simulink model "OpenLoopLinearSimulink"  (R2023a)
settings: Solver=VariableStepAuto  StartTime=0.0  StopTime=14  RelTol=1e-3
values from neighbouring files (symbols this model uses):
  contrDerivs = [-0.166531614792 0.0128973723454 19.613884709 0 0 15.5648221946 0 0 0.0210537390355 -0.0037893723417 -0.882539324975 9.80664666251 ... (1248 elements, 48x26)]    [contrDerivs.mat]
  V_vals = [1, 5, 10, 15, 20, 25, 30, 35, 40, 45, 50, 55, 60, 65,      70, 75, 80, 85, 90, 95, 100, 105, 110, 115, 120, 125]    [coaxial_heli_parameters.m]    (also in initializeCCH.m = [1, 5, 10, 15, 20, 25, 30, 35, 40, 45, 50, 55, 60, 65,      )
  ytrim = ytrim(:,ii)    [initLinCCH6dof.m]
undefined symbols (not defined in the file or in its folder): stabDerivs
libraries: simulink_extras x3, cstblocks x1
settings Model: Creator=prenc  LastModifiedBy=prenc

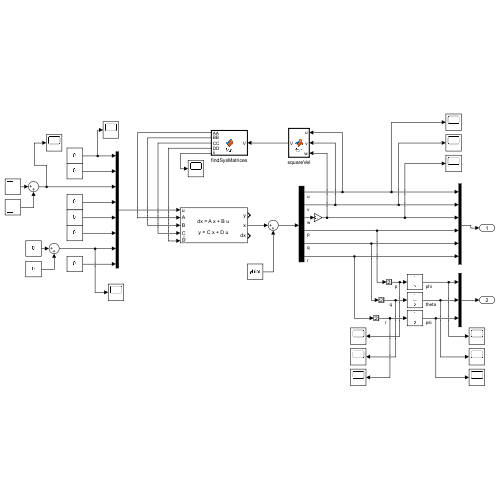
[thumbnail: Simulink's stored preview of the top-level diagram]
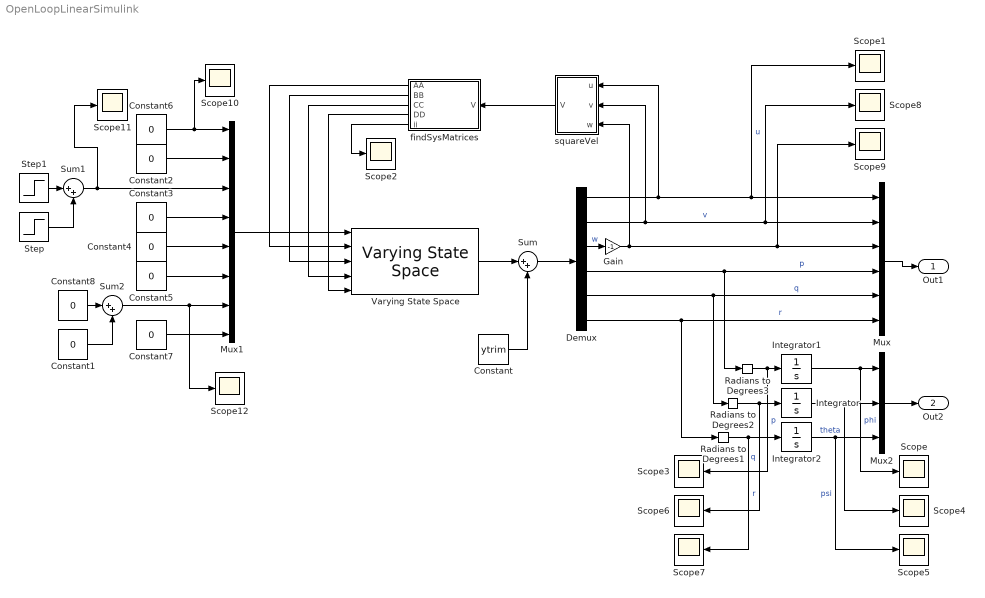
== system OpenLoopLinearSimulink ==
  Constant : Constant  Value=ytrim
  Constant{1..8} (8 alike) : Constant  Value=0
  Demux : Demux  Outputs=6
  Gain : Gain  Gain=-1
  Integrator : Integrator
  Integrator1 : Integrator
  Integrator2 : Integrator
  Mux : Mux  Inputs=6
  Mux1 : Mux  Inputs=8
  Mux2 : Mux  Inputs=3
  Radians to Degrees1 : simulink_extras/Transformations/Radians to Degrees
  Radians to Degrees2 : simulink_extras/Transformations/Radians to Degrees
  Radians to Degrees3 : simulink_extras/Transformations/Radians to Degrees
  Scope{,1..12} (13 alike) : Scope
  Step : Step  Time=4  After=deg2rad(1)  SampleTime=0
  Step1 : Step  Time=4.5  After=deg2rad(-1)  SampleTime=0
  Sum : Sum  Inputs=|++
  Sum1 : Sum  Inputs=|++
  Sum2 : Sum  Inputs=|++
  Varying State Space : cstblocks/Linear Parameter Varying/Varying State Space  x0=0  xNames=''  OutputX=on  OutputDX=on  Feedthrough=on
  findSysMatrices : MATLAB Function  TreatAsAtomicUnit=on
  squareVel : MATLAB Function  TreatAsAtomicUnit=on
  Out1 : Outport
  Out2 : Outport  Port=2
  wires:
  Demux/3 -> Gain/1  "w"
  Constant/1 -> Sum/2
  Demux/4 -> Radians to Degrees3/1, Mux/4  "p"
  Integrator2/1 -> Scope5/1, Mux2/3  "psi"
  Sum/1 -> Demux/1
  Demux/5 -> Radians to Degrees2/1, Mux/5  "q"
  Mux2/1 -> Out2/1
  Demux/2 -> Scope8/1, Mux/2, squareVel/2(v)  "v"
  Mux/1 -> Out1/1
  Mux1/1 -> Varying State Space/1
  Integrator/1 -> Scope4/1, Mux2/2  "theta"
  Demux/6 -> Radians to Degrees1/1, Mux/6  "r"
  Demux/1 -> Scope1/1, Mux/1, squareVel/1(u)  "u"
  Integrator1/1 -> Scope/1, Mux2/1  "phi"
  Constant6/1 -> Scope10/1, Mux1/1
  Constant2/1 -> Mux1/2
  Constant3/1 -> Mux1/4
  Constant4/1 -> Mux1/5
  Constant5/1 -> Mux1/6
  Sum2/1 -> Scope12/1, Mux1/7
  Constant7/1 -> Mux1/8
  Sum1/1 -> Scope11/1, Mux1/3
  Radians to Degrees2/1 -> Scope6/1, Integrator/1  "q"
  Radians to Degrees1/1 -> Scope7/1, Integrator2/1  "r"
  Radians to Degrees3/1 -> Scope3/1, Integrator1/1  "p"
  squareVel/1(V) -> findSysMatrices/1(V)
  findSysMatrices/2(BB) -> Varying State Space/3
  findSysMatrices/3(CC) -> Varying State Space/4
  findSysMatrices/4(DD) -> Varying State Space/5
  findSysMatrices/5(ii) -> Scope2/1
  findSysMatrices/1(AA) -> Varying State Space/2
  Varying State Space/2 -> Sum/1
  Gain/1 -> Scope9/1, Mux/3, squareVel/3(w)
  Constant1/1 -> Sum2/2
  Constant8/1 -> Sum2/1
  Step/1 -> Sum1/2
  Step1/1 -> Sum1/1

== matlab function OpenLoopLinearSimulink/squareVel ==
  data: u input; V output; v input; w input; trimvelocity parameter
function V = fcn(u,v,w, trimvelocity)

V = sqrt(u^2+v^2+w^2);

== matlab function OpenLoopLinearSimulink/findSysMatrices ==
  data: V input; AA output; BB output; CC output; DD output; V_vals parameter; stabDerivs parameter; contrDerivs parameter; ii output
function [AA, BB, CC, DD, ii] = fcn(V, V_vals, stabDerivs, contrDerivs)

    [~, ii] = min(abs(V_vals - V));
   

    X_u = stabDerivs(1,:); X_v = stabDerivs(2,:); X_w = stabDerivs(3,:); X_p = stabDerivs(4,:); X_q = stabDerivs(5,:); X_r = stabDerivs(6,:);
    Y_u = stabDerivs(7,:); Y_v = stabDerivs(8,:); Y_w = stabDerivs(9,:); Y_p = stabDerivs(10,:); Y_q = stabDerivs(11,:); Y_r = stabDerivs(12,:);
    Z_u = stabDerivs(13,:); Z_v = stabDerivs(14,:); Z_w = stabDerivs(15,:); Z_p = stabDerivs(16,:); Z_q = stabDerivs(17,:); Z_r = stabDerivs(18,:);
    L_u = stabDerivs(19,:); L_v = stabDerivs(20,:); L_w = stabDerivs(21,:); L_p = stabDerivs(22,:); L_q = stabDerivs(23,:); L_r = stabDerivs(24,:);
    M_u = stabDerivs(25,:); M_v = stabDerivs(26,:); M_w = stabDerivs(27,:); M_p = stabDerivs(28,:); M_q = stabDerivs(29,:); M_r = stabDerivs(30,:);
    N_u = stabDerivs(31,:); N_v = stabDerivs(32,:); N_w = stabDerivs(33,:); N_p = stabDerivs(34,:); N_q = stabDerivs(35,:); N_r = stabDerivs(36,:);

    
    AA = [X_u(ii), X_v(ii), X_w(ii), X_p(ii), X_q(ii), X_r(ii);
            Y_u(ii), Y_v(ii), Y_w(ii), Y_p(ii), Y_q(ii), Y_r(ii);
            Z_u(ii), Z_v(ii), Z_w(ii), Z_p(ii), Z_q(ii), Z_r(ii);
            L_u(ii), L_v(ii), L_w(ii), L_p(ii), L_q(ii), L_r(ii);
            M_u(ii), M_v(ii), M_w(ii), M_p(ii), M_q(ii), M_r(ii);
            N_u(ii), N_v(ii), N_w(ii), N_p(ii), N_q(ii), N_r(ii)];
    
    X_theta_0 = contrDerivs(1,:); X_theta_d = contrDerivs(2,:); X_theta_s = contrDerivs(3,:); X_theta_c = contrDerivs(4,:); X_theta_cdiff = contrDerivs(5,:); X_theta_p = contrDerivs(6,:); X_delta_e = contrDerivs(7,:); X_delta_r = contrDerivs(8,:);
    Y_theta_0 = contrDerivs(9,:); Y_theta_d = contrDerivs(10,:); Y_theta_s = contrDerivs(11,:); Y_theta_c = contrDerivs(12,:); Y_theta_cdiff = contrDerivs(13,:); Y_theta_p = contrDerivs(14,:); Y_delta_e = contrDerivs(15,:); Y_delta_r = contrDerivs(16,:);
    Z_theta_0 = contrDerivs(17,:); Z_theta_d = contrDerivs(18,:); Z_theta_s = contrDerivs(19,:); Z_theta_c = contrDerivs(20,:); Z_theta_cdiff = contrDerivs(21,:); Z_theta_p = contrDerivs(22,:); Z_delta_e = contrDerivs(23,:); Z_delta_r = contrDerivs(24,:);
    L_theta_0 = contrDerivs(25,:); L_theta_d = contrDerivs(26,:); L_theta_s = contrDerivs(27,:); L_theta_c = contrDerivs(28,:); L_theta_cdiff = contrDerivs(29,:); L_theta_p = contrDerivs(30,:); L_delta_e = contrDerivs(31,:); L_delta_r = contrDerivs(32,:);
    M_theta_0 = contrDerivs(33,:); M_theta_d = contrDerivs(34,:); M_theta_s = contrDerivs(35,:); M_theta_c = contrDerivs(36,:); M_theta_cdiff = contrDerivs(37,:); M_theta_p = contrDerivs(38,:); M_delta_e = contrDerivs(39,:); M_delta_r = contrDerivs(40,:);
    N_theta_0 = contrDerivs(41,:); N_theta_d = contrDerivs(42,:); N_theta_s = contrDerivs(43,:); N_theta_c = contrDerivs(44,:); N_theta_cdiff = contrDerivs(45,:); N_theta_p = contrDerivs(46,:); N_delta_e = contrDerivs(47,:); N_delta_r = contrDerivs(48,:);

    BB = [X_theta_0(ii), X_theta_d(ii), X_theta_s(ii), X_theta_c(ii), X_theta_cdiff(ii), X_theta_p(ii), X_delta_e(ii), X_delta_r(ii);
            Y_theta_0(ii), Y_theta_d(ii), Y_theta_s(ii), Y_theta_c(ii), Y_theta_cdiff(ii), Y_theta_p(ii), Y_delta_e(ii), Y_delta_r(ii);
            Z_theta_0(ii), Z_theta_d(ii), Z_theta_s(ii), Z_theta_c(ii), Z_theta_cdiff(ii), Z_theta_p(ii), Z_delta_e(ii), Z_delta_r(ii);
            L_theta_0(ii), L_theta_d(ii), L_theta_s(ii), L_theta_c(ii), L_theta_cdiff(ii), L_theta_p(ii), L_delta_e(ii), L_delta_r(ii);
            M_theta_0(ii), M_theta_d(ii), M_theta_s(ii), M_theta_c(ii), M_theta_cdiff(ii), M_theta_p(ii), M_delta_e(ii), M_delta_r(ii);
            N_theta_0(ii), N_theta_d(ii), N_theta_s(ii), N_theta_c(ii), N_theta_cdiff(ii), N_theta_p(ii), N_delta_e(ii), N_delta_r(ii)]; 

    CC = eye(size(AA));
    DD = zeros(size(BB));

end
